simulink model "sim_friction_model"  (R2015b)
settings: Solver=VariableStepAuto  StartTime=0.0  StopTime=10  FixedStep=0.001  RelTol=1e-3
values from neighbouring files (symbols this model uses):
  lin_sys_A = self.lin_system_par_struct.A    [Friction_model.m]
  lin_sys_B = self.lin_system_par_struct.B    [Friction_model.m]
  lin_sys_C = self.lin_system_par_struct.C    [Friction_model.m]
  lin_sys_D = self.lin_system_par_struct.D    [Friction_model.m]
  lin_sys_X = self.lin_system_par_struct.X    [Friction_model.m]
(part 1 of 2)
settings Model: Creator=dave  LastModifiedBy=dave

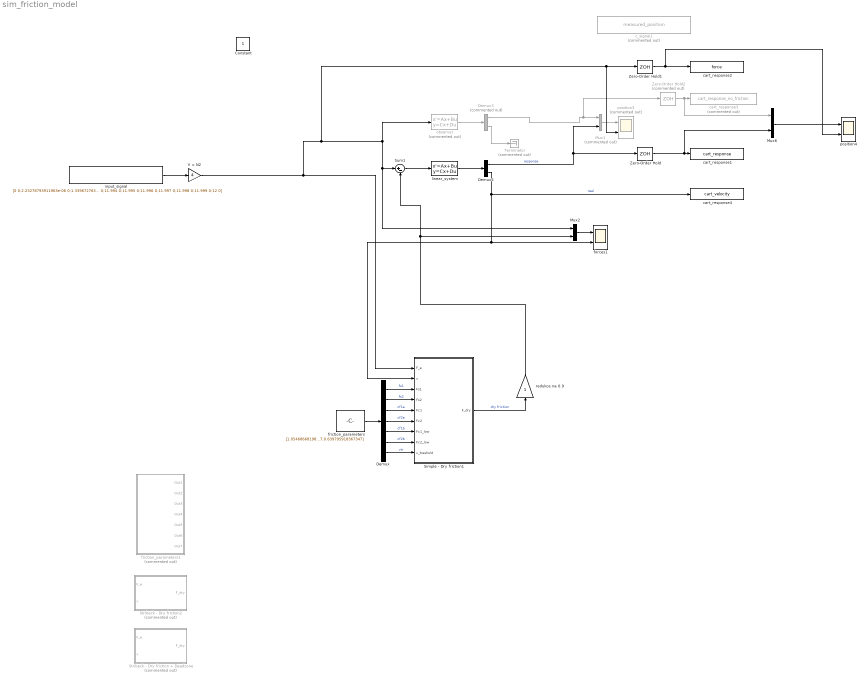
== system sim_friction_model ==
  Demux : Demux  Outputs=7
  Demux3 : Demux  Commented=on  Outputs=2
  Demux4 : Demux  Outputs=2
  Mux1 : Mux  Commented=on  Inputs=2
  Mux2 : Mux  Inputs=2
  Mux6 : Mux  Inputs=2
  Simple - Dry friction1 : MATLAB Function  TreatAsAtomicUnit=on
  Stribeck - Dry friction + Deadzone : MATLAB Function  Commented=on  TreatAsAtomicUnit=on
  Stribeck - Dry friction2 : MATLAB Function  Commented=on  TreatAsAtomicUnit=on
  Sum1 : Sum  Inputs=|+-
  Terminator : Terminator  Commented=on
  V > N2 : Gain  Gain=4
  Zero-Order Hold : ZeroOrderHold  SampleTime=0.001
  Zero-Order Hold1 : ZeroOrderHold  SampleTime=0.001
  Zero-Order Hold2 : ZeroOrderHold  Commented=on  SampleTime=0.001
  c_signal1 : FromWorkspace  Commented=on  VariableName=measured_position  SampleTime=0
  cart_response1 : ToWorkspace  VariableName=cart_response  SaveFormat=Timeseries  SampleTime=-1
  cart_response2 : ToWorkspace  VariableName=force  SaveFormat=Timeseries  SampleTime=-1
  cart_response3 : ToWorkspace  Commented=on  VariableName=cart_response_no_friction  SaveFormat=Timeseries  SampleTime=-1
  cart_response4 : ToWorkspace  VariableName=cart_velocity  SaveFormat=Timeseries  SampleTime=-1
  forces1 : Scope  NumInputPorts=2
  friction_parameters : Constant  Value=[1.05468668198236;0.637122644398882;0.169976262832451;0.447415708441727;0.579424414089966;0.28554418727097;0.639795918367347]
  friction_parameters1 : Subsystem  Commented=on
  input_signal : FromWorkspace  VariableName=[0 0;2.23278793911963e-06 0;1.33967276347178e-05 0;6.92164261127084e-05 0;0.000348314918502662 0;0.001 0;0.002 0;0.003 0;0.004 0;0.005 0;0.006 0;0.007 0;0.008 0;0.009 0;0.01 0;0.011 0;0.012 0;0.013 0;0.014 0;0.015 0;0.016 0;0.017 0;0.018 0;0.019 0;0.02 0;0.021 0;0.022 0;0.023 0;0.024 0;0.025 0;0.026 0;0.027 0;0.028 0;0.029 0;0.03 0;0.031 0;0.032 0;0.033 0;0.034 0;0.035 0;0.036 0;0.037 0;0.038 0;0.039 0;0.04 0;0.041 0;0.042 0;0.043 0;0.044 0;0.045 0;0.046 0;0.047 0;0.048 0;0.049 0;0.05 0;0.051 0;0.052 0;0.053 0;0.054 0;0.055 0;0.056 0;0.057 0;0.058 0;0.059 0;0.06 0;0.061 0;0.062 0;0.063 0;0.064 0;0.065 0;0.066 0;0.067 0;0.068 0;0.069 0;0.07 0;0.071 0;0.072 0;0.073 0;0.074 0;0.075 0;0.076 0;0.077 0;0.078 0;0.079 0;0.08 0;0.081 0;0.082 0;0.083 0;0.084 0;0.085 0;0.086 0;0.087 0;0.088 0;0.089 0;0.09 0;0.091 0;0.092 0;0.093 0;0.094 0;0.095 0;0.096 0;0.097 0;0.098 0;0.099 0;0.1 0;0.101 0;0.102 0;0.103 0;0.104 0;0.105 0;0.106 0;0.107 0;0.108 0;0.109 0;0.11 0;0.111 0;0.112 0;0.113 0;0.114 0;0.115 0;0.116 0;0.117 0;0.118 0;0.119 0;0.12 0;0.121 0;0.122 0;0.123 0;0.124 0;0.125 0;0.126 0;0.127 0;0.128 0;0.129 0;0.13 0;0.131 0;0.132 0;0.133 0;0.134 0;0.135 0;0.136 0;0.137 0;0.138 0;0.139 0;0.14 0;0.141 0;0.142 0;0.143 0;0.144 0;0.145 0;0.146 0;0.147 0;0.148 0;0.149 0;0.15 0;0.151 0;0.152 0;0.153 0;0.154 0;0.155 0;0.156 0;0.157 0;0.158 0;0.159 0;0.16 0;0.161 0;0.162 0;0.163 0;0.164 0;0.165 0;0.166 0;0.167 0;0.168 0;0.169 0;0.17 0;0.171 0;0.172 0;0.173 0;0.174 0;0.175 0;0.176 0;0.177 0;0.178 0;0.179 0;0.18 0;0.181 0;0.182 0;0.183 0;0.184 0;0.185 0;0.186 0;0.187 0;0.188 0;0.189 0;0.19 0;0.191 0;0.192 0;0.193 0;0.194 0;0.195 0;0.196 0;0.197 0;0.198 0;0.199 0;0.2 0;0.201 0;0.202 0;0.203 0;0.204 0;0.205 0;0.206 0;0.207 0;0.208 0;0.209 0;0.21 0;0.211 0;0.212 0;0.213 0;0.214 0;0.215 0;0.216 0;0.217 0;0.218 0;0.219 0;0.22 0;0.221 0;0.222 0;0.223 0;0.224 0;0.225 0;0.226 0;0.227 0;0.228 0;0.229 0;0.23 0;0.231 0;0.232 0;0.233 0;0.234 0;0.235 0;0.236 0;0.237 0;0.238 0;0.239 0;0.24 0;0.241 0;0.242 0;0.243 0;0.244 0;0.245 0;0.246 0;0.247 0;0.248 0;0.249 0;0.25 0;0.251 0;0.252 0;0.253 0;0.254 0;0.255 0;0.256 0;0.257 0;0.258 0;0.259 0;0.26 0;0.261 0;0.262 0;0.263 0;0.264 0;0.265 0;0.266 0;0.267 0;0.268 0;0.269 0;0.27 0;0.271 0;0.272 0;0.273 0;0.274 0;0.275 0;0.276 0;0.277 0;0.278 0;0.279 0;0.28 0;0.281 0;0.282 0;0.283 0;0.284 0;0.285 0;0.286 0;0.287 0;0.288 0;0.289 0;0.29 0;0.291 0;0.292 0;0.293 0;0.294 0;0.295 0;0.296 0;0.297 0;0.298 0;0.299 0;0.3 0;0.301 0;0.302 0;0.303 0;0.304 0;0.305 0;0.306 0;0.307 0;0.308 0;0.309 0;0.31 0;0.311 0;0.312 0;0.313 0;0.314 0;0.315 0;0.316 0;0.317 0;0.318 0;0.319 0;0.32 0;0.321 0;0.322 0;0.323 0;0.324 0;0.325 0;0.326 0;0.327 0;0.328 0;0.329 0;0.33 0;0.331 0;0.332 0;0.333 0;0.334 0;0.335 0;0.336 0;0.337 0;0.338 0;0.339 0;0.34 0;0.341 0;0.342 0;0.343 0;0.344 0;0.345 0;0.346 0;0.347 0;0.348 0;0.349 0;0.35 0;0.351 0;0.352 0;0.353 0;0.354 0;0.355 0;0.356 0;0.357 0;0.358 0;0.359 0;0.36 0;0.361 0;0.362 0;0.363 0;0.364 0;0.365 0;0.366 0;0.367 0;0.368 0;0.369 0;0.37 0;0.371 0;0.372 0;0.373 0;0.374 0;0.375 0;0.376 0;0.377 0;0.378 0;0.379 0;0.38 0;0.381 0;0.382 0;0.383 0;0.384 0;0.385 0;0.386 0;0.387 0;0.388 0;0.389 0;0.39 0;0.391 0;0.392 0;0.393 0;0.394 0;0.395 0;0.396 0;0.397 0;0.398 0;0.399 0;0.4 0;0.401 0;0.402 0;0.403 0;0.404 0;0.405 0;0.406 0;0.407 0;0.408 0;0.409 0;0.41 0;0.411 0;0.412 0;0.413 0;0.414 0;0.415 0;0.416 0;0.417 0;0.418 0;0.419 0;0.42 0;0.421 0;0.422 0;0.423 0;0.424 0;0.425 0;0.426 0;0.427 0;0.428 0;0.429 0;0.43 0;0.431 0;0.432 0;0.433 0;0.434 0;0.435 0;0.436 0;0.437 0;0.438 0;0.439 0;0.44 0;0.441 0;0.442 0;0.443 0;0.444 0;0.445 0;0.446 0;0.447 0;0.448 0;0.449 0;0.45 0;0.451 0;0.452 0;0.453 0;0.454 0;0.455 0;0.456 0;0.457 0;0.458 0;0.459 0;0.46 0;0.461 0;0.462 0;0.463 0;0.464 0;0.465 0;0.466 0;0.467 0;0.468 0;0.469 0;0.47 0;0.471 0;0.472 0;0.473 0;0.474 0;0.475 0;0.476 0;0.477 0;0.478 0;0.479 0;0.48 0;0.481 0;0.482 0;0.483 0;0.484 0;0.485 0;0.486 0;0.487 0;0.488 0;0.489 0;0.49 0;0.491 0;0.492 0;0.493 0;0.494 0 ...(+93184 chars)]  SampleTime=0
  linear_system : StateSpace  A=[0 1;0 -2.6]  B=[0;0.37037037037037]  C=[1 0;0 1]  D=[0;0]  X0=[0 0]
  observer : StateSpace  Commented=on  A=lin_sys_A  B=lin_sys_B  C=lin_sys_C  D=lin_sys_D  X0=lin_sys_X
  position3 : Scope  Commented=on  NumInputPorts=2
  position4 : Scope  NumInputPorts=2
  redukce na 0.9 : Gain
  Constant : Constant  IOType=siggen
  wires:
  Sum1/1 -> linear_system/1
  observer/1 -> Demux3/1
  linear_system/1 -> Demux4/1
  Demux4/2 -> forces1/2, Simple - Dry friction1/2(v), cart_response4/1  "real"
  Mux2/1 -> forces1/1
  Simple - Dry friction1/1(F_dry) -> redukce na 0.9/1  "dry friction"
  Demux4/1 -> Mux1/2, Zero-Order Hold/1  "response"
  Demux3/2 -> Terminator/1
  Zero-Order Hold1/1 -> position4/2, cart_response2/1
  Demux3/1 -> Zero-Order Hold2/1, Mux1/1
  Mux1/1 -> position3/1
  Zero-Order Hold2/1 -> Mux6/1, cart_response3/1
  redukce na 0.9/1 -> Mux2/2, Sum1/2
  Mux6/1 -> position4/1
  input_signal/1 -> V > N2/1
  Zero-Order Hold/1 -> Mux6/2, cart_response1/1
  V > N2/1 -> Simple - Dry friction1/1(F_e), position3/2, Zero-Order Hold1/1, observer/1, Mux2/1, Sum1/1
  Demux/1 -> Simple - Dry friction1/3(Fs1)  "fs1"
  Demux/2 -> Simple - Dry friction1/4(Fs2)  "fs2"
  Demux/3 -> Simple - Dry friction1/5(Fc1)  "cf1a"
  Demux/4 -> Simple - Dry friction1/6(Fc2)  "cf2a"
  Demux/5 -> Simple - Dry friction1/7(Fc1_low)  "cf1b"
  Demux/6 -> Simple - Dry friction1/8(Fc2_low)  "cf2b"
  Demux/7 -> Simple - Dry friction1/9(v_treshold)  "vtr"
  friction_parameters/1 -> Demux/1
